simulink model "Lab_1"  (Simulink 9.1)
settings: Solver=ode45  StartTime=0.0  StopTime=10  RelTol=1e-7
values from neighbouring files (symbols this model uses):
  I = [I_1,   0,  0 ... (first row only)    [main.m]
  I_inv = inv(I)    [main.m]
  w_0 = [w1_0, w2_0, w3_0]    [main.m]
libraries: sharedutil x1
settings Model: SuppressorTable=22 serialization::archive 11 0 6 0 0 0 1 0  Creator=fcuzzocrea  LastModifiedBy=fcuzzocrea
settings DataIOCC: SaveFormat=Dataset
settings OptimizationCC: LifeSpan=auto
settings DebuggingCC: UnderspecifiedInitializationDetection=Simplified  MergeDetectMultiDrivingBlocksExec=error  SFUnexpectedBacktrackingDiag=error  SFNoUnconditionalDefaultTransitionDiag=error  SFExecutionAtInitializationDiag=warning
settings HardwareCC: ProdBitPerPointer=64  ProdBitPerSizeT=64  ProdBitPerPtrDiffT=64  ProdLargestAtomicFloat=Float  ProdIntDivRoundTo=Zero  ProdEndianess=LittleEndian  ProdWordSize=64  ProdHWDeviceType=Intel->x86-64 (Windows64)
settings ModelReferenceCC: PropagateSignalLabelsOutOfModel=on
settings CodeAppCC: StateflowObjectComments=off
settings GRTTargetCC: TargetLangStandard=C99 (ISO)  CombineOutputUpdateFcns=on  GRTInterface=off
settings ConfigComp: CovMetricSettings=dwe  CovHtmlReporting=off  CovSaveCumulativeToWorkspaceVar=off  CovSaveSingleToWorkspaceVar=off  CovExternalEMLEnable=on

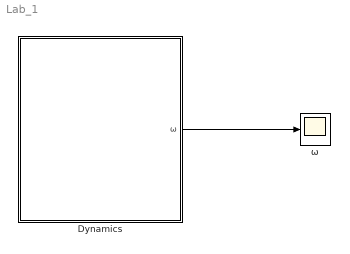
== system Lab_1 ==
  "Dynamics  " : Subsystem
  "ω " : Scope
  wires:
  "Dynamics  "/1(ω) -> "ω "/1

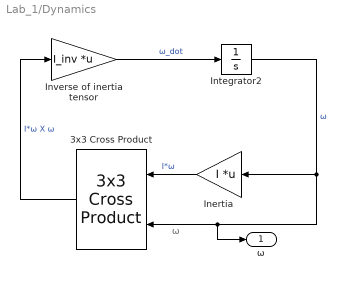
== system Lab_1/Dynamics   ==
  note: ω
  3x3 Cross Product : sharedutil/3x3 Cross Product  aMode=aMode
      settings: SourceProductBaseCode=AE
  Inertia : Gain  Gain=I  Multiplication=Matrix(K*u)
  Integrator2 : Integrator  InitialCondition=w_0
  Inverse of inertia tensor : Gain  Gain=I_inv  Multiplication=Matrix(K*u)
  ω : Outport
  wires:
  3x3 Cross Product/1 -> Inverse of inertia tensor/1  "I*ω X ω"
  Inertia/1 -> 3x3 Cross Product/1  "I*ω"
  Inverse of inertia tensor/1 -> Integrator2/1  "ω_dot"
  Integrator2/1 -> ω/1, 3x3 Cross Product/2, Inertia/1  "ω"
